simulink model "akh_rev_project"  (R2020b)
settings: Solver=ode45  StartTime=0.0  StopTime=10  FixedStep=Ts_Power  RelTol=1e-3  AbsTol=1e-2
InitFcn:
  | Fnom = 50;        % Hz
  | 
  | Fc = 27*Fnom;   % (Hz)
  | Ts_Power = 1/(Fc*100);
  | Ts_Control = Ts_Power*10;
values from neighbouring files (symbols this model uses):
  Ts = 1/fs    (= 1e-05)    [PE_46.m]    (also in disc_sim.m = 1; mass_spring_damper_model.m = 0.1)
undefined symbols (not defined in the file or in its folder): D1, D11, Delta, DiscIntNeverNeededParam, j, magnitude
libraries: powerlib x146, powerlib_meascontrol x90, simulink x2, re_lib x1
(part 2 of 8)

== system akh_rev_project/Source ==
  note: Adding negative-sequence and zero-sequence
      | 1 sec <  t < 1.5 sec
  note: Positive-sequence magnitude variation
  note: Vabc
      | Frequency Modulation
      |  58 /62 Hz
      |  Freq=1 Hz
  note: t = 1.75 sec
      | phase variation:
      | delta_phase= -60 deg
  note: t> 2 sec
      | Ajout d'harmoniques
      |  20% 3e  seq homopolaire
      |  30%  4e  seq directe
  -180 < alpha < 180 : Subsystem
  Bus Selector : BusSelector  OutputSignals=Freq (Hz)
  Bus Selector1 : BusSelector  OutputSignals=wt (rad)
  Mag (pu)2 : powerlib_meascontrol/Pulse & Signal Generators/Stair Generator  t="[0, 0.2, 0.3,  1]"  e="[1, 0.0,  1,  1.2]"  Ts=Ts
  Step : Step  Time=1.75  After=-90  SampleTime=0
  Sum : Sum  Inputs=+++
  Sum1 : Sum  Inputs=+-
  Synchronous Reference : powerlib_meascontrol/Pulse & Signal Generators/Three-Phase Programmable Generator  Par_Vps=[1, 0 , 60]  VariationEntity=None  VariationType=Modulation  VariationStep=-0.5  VariationRate=10  VariationMag=2  VariationFreq=1  Par_Timing_Variation="[0.5  99]"  SinglePhase=on  Yampli=[1 0.2 1.2 1.0]  Xtime=[0 0.1 0.15 0.2]  HarmonicGeneration=off  Par_HarmoA="[1  0.5  -25  0]"  Par_HarmoB="[1  0.1  35  2]"  Par_Timing_Harmo=[ 1 99]  Ts=Ts
      settings: SourceProductBaseCode=PS
  Terminator{,1..3} (4 alike) : Terminator
  Three-Phase Programmable Generator : powerlib_meascontrol/Pulse & Signal Generators/Three-Phase Programmable Generator  Par_Vps=[1, 0 , 60]  VariationEntity=Frequency  VariationType=Modulation  VariationStep=-0.5  VariationRate=10  VariationMag=2  VariationFreq=1  Par_Timing_Variation="[0.5  99]"  SinglePhase=on  Yampli=[1 0.2 1.2 1.0]  Xtime=[0 0.1 0.15 0.2]  HarmonicGeneration=off  Par_HarmoA="[1  0.5  -25  0]"  Par_HarmoB="[1  0.1  35  2]"  Par_Timing_Harmo=[ 1 99]  Ts=Ts
      settings: SourceProductBaseCode=PS
  Three-Phase Programmable Generator1 : powerlib_meascontrol/Pulse & Signal Generators/Three-Phase Programmable Generator  Par_Vps=[0 , 0 , 60]  VariationEntity=Frequency  VariationType=Modulation  VariationStep=-0.5  VariationRate=10  VariationMag=2  VariationFreq=1  Par_Timing_Variation="[0.5  99]"  SinglePhase=on  Yampli=[1 0.2 1.2 1.0]  Xtime=[0 0.1 0.15 0.2]  HarmonicGeneration=on  Par_HarmoA="[1  0.4  90  2]"  Par_HarmoB="[1  0.3  35  0]"  Par_Timing_Harmo=[1 1.5]  Ts=Ts
      settings: SourceProductBaseCode=PS
  Three-Phase Programmable Generator2 : powerlib_meascontrol/Pulse & Signal Generators/Three-Phase Programmable Generator  Par_Vps=[0 , 0 , 60]  VariationEntity=Frequency  VariationType=Modulation  VariationStep=-0.5  VariationRate=10  VariationMag=2  VariationFreq=1  Par_Timing_Variation="[0.5  99]"  SinglePhase=on  Yampli=[1 0.2 1.2 1.0]  Xtime=[0 0.1 0.15 0.2]  HarmonicGeneration=on  Par_HarmoA="[3  0.2  0  0]"  Par_HarmoB="[4  0.3  60  1]"  Par_Timing_Harmo="[ 2  99]"  Ts=Ts
      settings: SourceProductBaseCode=PS
  Three-Phase Sine Generator : powerlib_meascontrol/Pulse & Signal Generators/Three-Phase Sine Generator  Ts=Ts
      settings: SourceProductBaseCode=PS
  Vabc : Outport  VectorParamsAs1DForOutWhenUnconnected=off
  angle(deg) : Outport  Port=2  VectorParamsAs1DForOutWhenUnconnected=off
  tag scope: Freq_ref=global, Mag_ref=global
  wires:
  Step/1 -> Three-Phase Sine Generator/2
  Three-Phase Programmable Generator/2 -> Bus Selector/1
  Bus Selector/1 -> Three-Phase Sine Generator/3, [Freq_ref]  "<Freq (Hz)>"
  Mag (pu)2/1 -> [Mag_ref], Three-Phase Sine Generator/1
  Three-Phase Programmable Generator1/1 -> Sum/2
  Sum/1 -> Vabc/1  "Vabc (pu)"
  Three-Phase Programmable Generator2/1 -> Sum/3
  Three-Phase Sine Generator/1 -> Sum/1
  Three-Phase Programmable Generator/1 -> Terminator/1
  Three-Phase Programmable Generator2/2 -> Terminator1/1
  Three-Phase Programmable Generator1/2 -> Terminator2/1
  Bus Selector1/1 -> Sum1/2  "<wt (rad)>"
  Sum1/1 -> -180 < alpha < 180/1(angle (rad))
  Synchronous Reference/2 -> Bus Selector1/1
  Three-Phase Sine Generator/2 -> Sum1/1
  Synchronous Reference/1 -> Terminator3/1
  -180 < alpha < 180/1(angle(deg)) -> angle(deg)/1

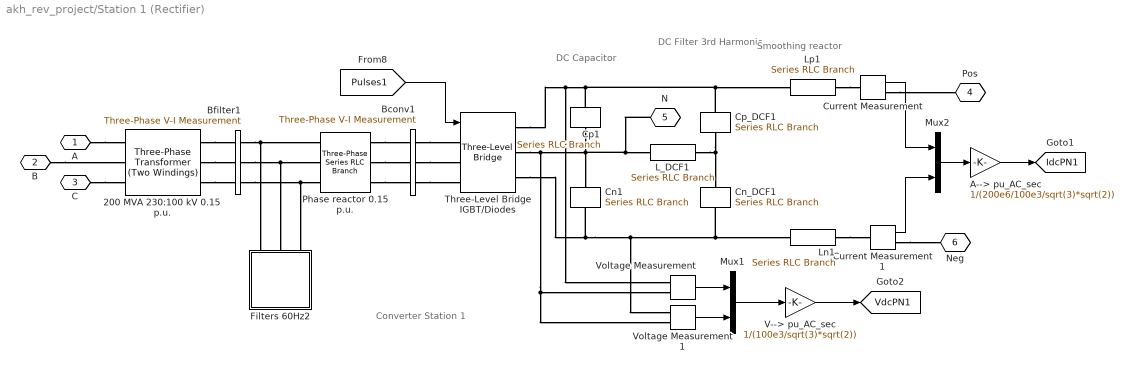
== system akh_rev_project/Station 1 (Rectifier) ==
  note: DC Capacitor
  note: Converter Station 1
  note: DC Filter
      | 3rd Harmonic
  note: Smoothing reactor
  200 MVA 230:100 kV 0.15 p.u. : powerlib/Elements/Three-Phase Transformer (Two Windings)  Winding1Connection=Yg  Winding2Connection=Delta (D1)  CoreType=Three single-phase transformers  SetSaturation=off  Hysteresis=off  DataFile='hysteresis'  SetInitialFlux=off  Measurements=None  UNITS=pu  NominalPower=[200e6 , Fnom]  Winding1="[230e3 * 0.915  0.0025 0.075]"  Winding2="[100e3  0.0025  0.075]"  Rm=500  Lm=500  L0=0.5  Saturation=[ 0,0 ; 0.012,1.25 ; 1.012,1.6 ]  InitialFluxes=[-1.03850588171453 0.527233233676132 0.511272648041703]  BreakLoop=off  DiscreteSolver=Trapezoidal iterative  DataType=off  TransfoNumber=0
  A--> pu_AC_sec : Gain  Gain=1/(200e6/100e3/sqrt(3)*sqrt(2))
  Bconv1 : powerlib/Measurements/Three-Phase V-I Measurement  VoltageMeasurement=phase-to-ground  SetLabelV=on  LabelV=Uv_abc1  Vpu=on  VpuLL=off  CurrentMeasurement=yes  SetLabelI=on  LabelI=Iv_abc1  Ipu=on  Pbase=200e6  Vbase=100e3  OutputType=Complex  PhasorSimulation=off  PSBequivalent=0
  Bfilter1 : powerlib/Measurements/Three-Phase V-I Measurement  VoltageMeasurement=phase-to-ground  SetLabelV=on  LabelV=Uf_abc1  Vpu=on  VpuLL=off  CurrentMeasurement=no  SetLabelI=off  LabelI=Iabc  Ipu=off  Pbase=100e6  Vbase=100e3  OutputType=Complex  PhasorSimulation=off  PSBequivalent=0
  Cn1 : powerlib/Elements/Series RLC Branch  LConnTagsString=__new0  RConnTagsString=__new0  BranchType=C  Resistance=[]  Inductance=[]  SetiL0=off  InitialCurrent=0  Capacitance=70e-6  Setx0=off  InitialVoltage=0  Measurements=None
  Cn_DCF1 : powerlib/Elements/Series RLC Branch  LConnTagsString=__new0  RConnTagsString=__new0  BranchType=C  Resistance=[]  Inductance=[]  SetiL0=off  InitialCurrent=0  Capacitance=12e-6  Setx0=off  InitialVoltage=0  Measurements=None
  Cp1 : powerlib/Elements/Series RLC Branch  LConnTagsString=__new0  RConnTagsString=__new0  BranchType=C  Resistance=[]  Inductance=[]  SetiL0=off  InitialCurrent=0  Capacitance=70e-6  Setx0=off  InitialVoltage=0  Measurements=None
  Cp_DCF1 : powerlib/Elements/Series RLC Branch  LConnTagsString=__new0  RConnTagsString=__new0  BranchType=C  Resistance=[]  Inductance=[]  SetiL0=off  InitialCurrent=0  Capacitance=12e-6  Setx0=off  InitialVoltage=0  Measurements=None
  Current Measurement : powerlib/Measurements/Current Measurement  PhasorSimulation=off  OutputType=Complex  PSBequivalent=0
  Current Measurement1 : powerlib/Measurements/Current Measurement  PhasorSimulation=off  OutputType=Complex  PSBequivalent=0
  Filters 60Hz2 : Subsystem
      mask Display: disp('AC filters\n40 Mvar')
  L_DCF1 : powerlib/Elements/Series RLC Branch  LConnTagsString=__new0  RConnTagsString=__new0  BranchType=RL  Resistance=0.14737  Inductance=46.908e-3  SetiL0=off  InitialCurrent=0  Capacitance=[]  Setx0=off  InitialVoltage=0  Measurements=None
  Ln1 : powerlib/Elements/Series RLC Branch  LConnTagsString=__new0  RConnTagsString=__new0  BranchType=RL  Resistance=0.0251  Inductance=8.0e-3  SetiL0=off  InitialCurrent=0  Capacitance=[]  Setx0=off  InitialVoltage=0  Measurements=Branch current
  Lp1 : powerlib/Elements/Series RLC Branch  LConnTagsString=__new0  RConnTagsString=__new0  BranchType=RL  Resistance=0.0251  Inductance=8.0e-3  SetiL0=off  InitialCurrent=0  Capacitance=[]  Setx0=off  InitialVoltage=0  Measurements=Branch current
  Mux1 : Mux  Inputs=2
  Mux2 : Mux  Inputs=2
  Phase reactor 0.15 p.u. : powerlib/Elements/Three-Phase Series RLC Branch  LConnTagsString=A|B|C  RConnTagsString=A|B|C  BranchType=RL  Resistance=0.0015*(100^2 / 200)  Inductance=0.15* (100^2 / 200) / (2*pi*Fnom)  Capacitance=1.0  Measurements=None
  Three-Level Bridge IGBT/Diodes : powerlib/Power Electronics/Three-Level Bridge  Arms=3  SnubberResistance=5000  SbubberCapacitance=1e-6  Device=IGBT / Diodes  Ron=1e-3  ForwardVoltages="[  0  0  ]"  Measurements=None
      settings: SourceProductBaseCode=PS
  V--> pu_AC_sec : Gain  Gain=1/(100e3/sqrt(3)*sqrt(2))
  Voltage Measurement : powerlib/Measurements/Voltage Measurement  PhasorSimulation=off  OutputType=Complex  PSBequivalent=0
  Voltage Measurement1 : powerlib/Measurements/Voltage Measurement  PhasorSimulation=off  OutputType=Complex  PSBequivalent=0
  A : PMIOPort  Side=Left
  B : PMIOPort  Port=2  Side=Left
  C : PMIOPort  Port=3  Side=Left
  Pos : PMIOPort  Tag=PMCPort  Port=4  Side=Right
  N : PMIOPort  Tag=PMCPort  Port=5  Side=Right
  Neg : PMIOPort  Tag=PMCPort  Port=6  Side=Right
  tag scope: IdcPN1=global, VdcPN1=global
  wires:
  [Pulses1] -> Three-Level Bridge IGBT/Diodes/1
  Current Measurement/1 -> Mux2/1
  Current Measurement1/1 -> Mux2/2
  Mux2/1 -> A--> pu_AC_sec/1
  Voltage Measurement/1 -> Mux1/1
  Voltage Measurement1/1 -> Mux1/2
  Mux1/1 -> V--> pu_AC_sec/1
  V--> pu_AC_sec/1 -> [VdcPN1]
  A--> pu_AC_sec/1 -> [IdcPN1]
  connections:
  A/RConn1 -- 200 MVA 230:100 kV 0.15 p.u./LConn1
  B/RConn1 -- 200 MVA 230:100 kV 0.15 p.u./LConn2
  C/RConn1 -- 200 MVA 230:100 kV 0.15 p.u./LConn3
  Phase reactor 0.15 p.u./RConn1 -- Bconv1/LConn1
  Phase reactor 0.15 p.u./RConn2 -- Bconv1/LConn2
  Phase reactor 0.15 p.u./RConn3 -- Bconv1/LConn3
  Bconv1/RConn1 -- Three-Level Bridge IGBT/Diodes/LConn1
  Bconv1/RConn2 -- Three-Level Bridge IGBT/Diodes/LConn2
  Bconv1/RConn3 -- Three-Level Bridge IGBT/Diodes/LConn3
  Cn1/RConn1 -- Three-Level Bridge IGBT/Diodes/RConn3 -- Voltage Measurement1/LConn1 -- Cn_DCF1/RConn1 -- Ln1/LConn1
  Cp_DCF1/LConn1 -- Three-Level Bridge IGBT/Diodes/RConn1 -- Voltage Measurement/LConn1 -- Cp1/LConn1 -- Lp1/LConn1
  Current Measurement/RConn1 -- Pos/RConn1
  Current Measurement1/RConn1 -- Neg/RConn1
  200 MVA 230:100 kV 0.15 p.u./RConn1 -- Bfilter1/LConn1
  200 MVA 230:100 kV 0.15 p.u./RConn2 -- Bfilter1/LConn2
  200 MVA 230:100 kV 0.15 p.u./RConn3 -- Bfilter1/LConn3
  Bfilter1/RConn2 -- Phase reactor 0.15 p.u./LConn2 -- Filters 60Hz2/LConn2
  Bfilter1/RConn3 -- Phase reactor 0.15 p.u./LConn3 -- Filters 60Hz2/LConn3
  Bfilter1/RConn1 -- Phase reactor 0.15 p.u./LConn1 -- Filters 60Hz2/LConn1
  Cp_DCF1/RConn1 -- Cn_DCF1/LConn1 -- L_DCF1/RConn1
  N/RConn1 -- Voltage Measurement/LConn2 -- Voltage Measurement1/LConn2 -- Three-Level Bridge IGBT/Diodes/RConn2 -- Cn1/LConn1 -- Cp1/RConn1 -- L_DCF1/LConn1
  Lp1/RConn1 -- Current Measurement/LConn1
  Ln1/RConn1 -- Current Measurement1/LConn1

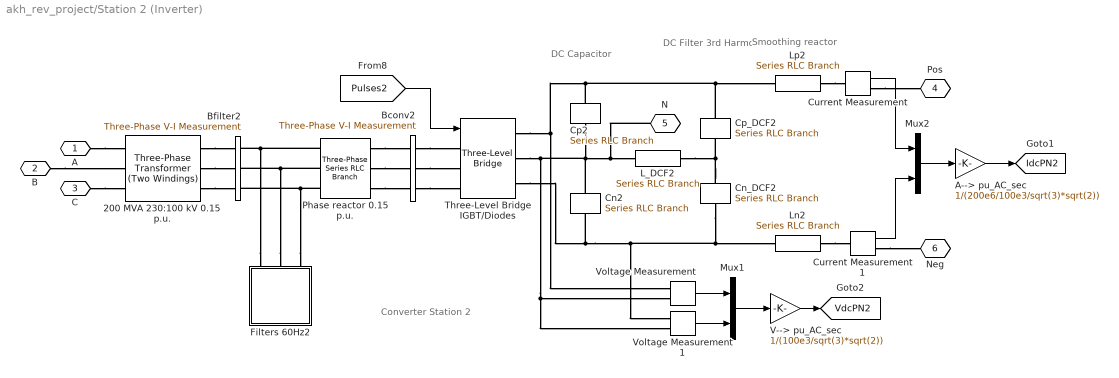
== system akh_rev_project/Station 2 (Inverter) ==
  note: Converter Station 2
  note: DC Capacitor
  note: DC Filter
      | 3rd Harmonic
  note: Smoothing reactor
  200 MVA 230:100 kV 0.15 p.u. : powerlib/Elements/Three-Phase Transformer (Two Windings)  Winding1Connection=Yg  Winding2Connection=Delta (D1)  CoreType=Three single-phase transformers  SetSaturation=off  Hysteresis=off  DataFile='hysteresis'  SetInitialFlux=off  Measurements=None  UNITS=pu  NominalPower=[200e6 , Fnom]  Winding1="[230e3 * 1.015   0.0025  0.075]"  Winding2="[100e3  0.0025  0.075]"  Rm=500  Lm=500  L0=0.5  Saturation=[ 0,0 ; 0.012,1.25 ; 1.012,1.6 ]  InitialFluxes=[-1.00735070526646 0.511416236666093 0.495934468600514]  BreakLoop=off  DiscreteSolver=Trapezoidal iterative  DataType=off  TransfoNumber=0
  A--> pu_AC_sec : Gain  Gain=1/(200e6/100e3/sqrt(3)*sqrt(2))
  Bconv2 : powerlib/Measurements/Three-Phase V-I Measurement  VoltageMeasurement=phase-to-ground  SetLabelV=on  LabelV=Uv_abc2  Vpu=on  VpuLL=off  CurrentMeasurement=yes  SetLabelI=on  LabelI=Iv_abc2  Ipu=on  Pbase=200e6  Vbase=100e3  OutputType=Complex  PhasorSimulation=off  PSBequivalent=0
  Bfilter2 : powerlib/Measurements/Three-Phase V-I Measurement  VoltageMeasurement=phase-to-ground  SetLabelV=on  LabelV=Uf_abc2  Vpu=on  VpuLL=off  CurrentMeasurement=no  SetLabelI=off  LabelI=Iabc  Ipu=off  Pbase=100e6  Vbase=100e3  OutputType=Complex  PhasorSimulation=off  PSBequivalent=0
  Cn2 : powerlib/Elements/Series RLC Branch  LConnTagsString=__new0  RConnTagsString=__new0  BranchType=C  Resistance=[]  Inductance=[]  SetiL0=off  InitialCurrent=0  Capacitance=70e-6  Setx0=off  InitialVoltage=0  Measurements=None
  Cn_DCF2 : powerlib/Elements/Series RLC Branch  LConnTagsString=__new0  RConnTagsString=__new0  BranchType=C  Resistance=[]  Inductance=[]  SetiL0=off  InitialCurrent=0  Capacitance=12e-6  Setx0=off  InitialVoltage=0  Measurements=None
  Cp2 : powerlib/Elements/Series RLC Branch  LConnTagsString=__new0  RConnTagsString=__new0  BranchType=C  Resistance=[]  Inductance=[]  SetiL0=off  InitialCurrent=0  Capacitance=70e-6  Setx0=off  InitialVoltage=0  Measurements=None
  Cp_DCF2 : powerlib/Elements/Series RLC Branch  LConnTagsString=__new0  RConnTagsString=__new0  BranchType=C  Resistance=[]  Inductance=[]  SetiL0=off  InitialCurrent=0  Capacitance=12e-6  Setx0=off  InitialVoltage=0  Measurements=None
  Current Measurement : powerlib/Measurements/Current Measurement  PhasorSimulation=off  OutputType=Complex  PSBequivalent=0
  Current Measurement1 : powerlib/Measurements/Current Measurement  PhasorSimulation=off  OutputType=Complex  PSBequivalent=0
  Filters 60Hz2 : Subsystem
      mask Display: disp('AC filters\n40 Mvar')
  L_DCF2 : powerlib/Elements/Series RLC Branch  LConnTagsString=__new0  RConnTagsString=__new0  BranchType=RL  Resistance=0.14737  Inductance=46.908e-3  SetiL0=off  InitialCurrent=0  Capacitance=[]  Setx0=off  InitialVoltage=0  Measurements=None
  Ln2 : powerlib/Elements/Series RLC Branch  LConnTagsString=__new0  RConnTagsString=__new0  BranchType=RL  Resistance=0.0251  Inductance=8.0e-3  SetiL0=off  InitialCurrent=0  Capacitance=[]  Setx0=off  InitialVoltage=0  Measurements=Branch current
  Lp2 : powerlib/Elements/Series RLC Branch  LConnTagsString=__new0  RConnTagsString=__new0  BranchType=RL  Resistance=0.0251  Inductance=8.0e-3  SetiL0=off  InitialCurrent=0  Capacitance=[]  Setx0=off  InitialVoltage=0  Measurements=Branch current
  Mux1 : Mux  Inputs=2
  Mux2 : Mux  Inputs=2
  Phase reactor 0.15 p.u. : powerlib/Elements/Three-Phase Series RLC Branch  LConnTagsString=A|B|C  RConnTagsString=A|B|C  BranchType=RL  Resistance=(0.15/100)*(100^2 / 200)  Inductance=0.15 * (100^2 / 200) / (2*pi*Fnom)  Capacitance=1.0  Measurements=None
  Three-Level Bridge IGBT/Diodes : powerlib/Power Electronics/Three-Level Bridge  Arms=3  SnubberResistance=5000  SbubberCapacitance=1e-6  Device=IGBT / Diodes  Ron=1e-3  ForwardVoltages="[ 0  0  ]"  Measurements=None
      settings: SourceProductBaseCode=PS
  V--> pu_AC_sec : Gain  Gain=1/(100e3/sqrt(3)*sqrt(2))
  Voltage Measurement : powerlib/Measurements/Voltage Measurement  PhasorSimulation=off  OutputType=Complex  PSBequivalent=0
  Voltage Measurement1 : powerlib/Measurements/Voltage Measurement  PhasorSimulation=off  OutputType=Complex  PSBequivalent=0
  A : PMIOPort  Side=Left
  B : PMIOPort  Port=2  Side=Left
  C : PMIOPort  Port=3  Side=Left
  Pos : PMIOPort  Tag=PMCPort  Port=4  Side=Right
  N : PMIOPort  Tag=PMCPort  Port=5  Side=Right
  Neg : PMIOPort  Tag=PMCPort  Port=6  Side=Right
  tag scope: IdcPN2=global, VdcPN2=global
  wires:
  Mux1/1 -> V--> pu_AC_sec/1
  Voltage Measurement1/1 -> Mux1/2
  Voltage Measurement/1 -> Mux1/1
  Mux2/1 -> A--> pu_AC_sec/1
  Current Measurement1/1 -> Mux2/2
  Current Measurement/1 -> Mux2/1
  [Pulses2] -> Three-Level Bridge IGBT/Diodes/1
  A--> pu_AC_sec/1 -> [IdcPN2]
  V--> pu_AC_sec/1 -> [VdcPN2]
  connections:
  Filters 60Hz2/LConn1 -- Bfilter2/RConn1 -- Phase reactor 0.15 p.u./LConn1
  Filters 60Hz2/LConn3 -- Bfilter2/RConn3 -- Phase reactor 0.15 p.u./LConn3
  Filters 60Hz2/LConn2 -- Bfilter2/RConn2 -- Phase reactor 0.15 p.u./LConn2
  200 MVA 230:100 kV 0.15 p.u./RConn3 -- Bfilter2/LConn3
  200 MVA 230:100 kV 0.15 p.u./RConn2 -- Bfilter2/LConn2
  200 MVA 230:100 kV 0.15 p.u./RConn1 -- Bfilter2/LConn1
  Current Measurement1/RConn1 -- Neg/RConn1
  Current Measurement/RConn1 -- Pos/RConn1
  Cp_DCF2/LConn1 -- Three-Level Bridge IGBT/Diodes/RConn1 -- Voltage Measurement/LConn1 -- Cp2/LConn1 -- Lp2/LConn1
  Cn_DCF2/RConn1 -- Voltage Measurement1/LConn1 -- Three-Level Bridge IGBT/Diodes/RConn3 -- Cn2/RConn1 -- Ln2/LConn1
  Cn2/LConn1 -- Voltage Measurement1/LConn2 -- Voltage Measurement/LConn2 -- Three-Level Bridge IGBT/Diodes/RConn2 -- Cp2/RConn1 -- L_DCF2/LConn1 -- N/RConn1
  Bconv2/RConn3 -- Three-Level Bridge IGBT/Diodes/LConn3
  Bconv2/RConn2 -- Three-Level Bridge IGBT/Diodes/LConn2
  Bconv2/RConn1 -- Three-Level Bridge IGBT/Diodes/LConn1
  Phase reactor 0.15 p.u./RConn3 -- Bconv2/LConn3
  Phase reactor 0.15 p.u./RConn2 -- Bconv2/LConn2
  Phase reactor 0.15 p.u./RConn1 -- Bconv2/LConn1
  C/RConn1 -- 200 MVA 230:100 kV 0.15 p.u./LConn3
  B/RConn1 -- 200 MVA 230:100 kV 0.15 p.u./LConn2
  A/RConn1 -- 200 MVA 230:100 kV 0.15 p.u./LConn1
  Cn_DCF2/LConn1 -- Cp_DCF2/RConn1 -- L_DCF2/RConn1
  Lp2/RConn1 -- Current Measurement/LConn1
  Ln2/RConn1 -- Current Measurement1/LConn1

== system akh_rev_project/VSC Controller Station 1 ==
  note: |-----------------------Ts_Control-----------------------|
  note: |------------Ts_Power------------|
  note: Sample time:
  note: |----------------Ts_Power--------------|
  note: Reference Steps
  note: VSC Controller
      | (Station 1)
  Anti-aliasing Filters : Subsystem  mask(Anti-aliasing (2nd order lowpass)){f0_aa=2000, Ts=Ts_Power}
      mask prompts: f0_aa "Cut-off frequency (Hz):"; Ts "Sample time:"
      mask init:
      | zeta = 1/sqrt(2);
  Block : Step  Time=0.3  Before=1  After=0  SampleTime=Ts_Control
  Constant1 : Constant  Value=0
  Constant2 : Constant  Value=0
  Constant3 : Constant  Value=1.0
  "Discrete VSC Controller " : Subsystem  mask(Discrete VSC-Based HVDC Controller){Mode=Active & Reactive Power, Xnom=[230e3, 100e3, Fnom, 200e3, 200e6], XP=[20.0, 1.0, -1.0, 1.43], Xdvco=[3.0, 3.0, 1.05, 0.9], XUdc=[2.0, 40.0 ], XQ=[20.0, 0.5, -0.5], Xvco=[3.0, 3.0, 1.05, 0.94], Xcrc=[1.1,  0.8], Xaccc=[0.6, 6.0,  0.3], enable_dcvbc=off, Xdcvbc=[0.2, 0.03], Ts_Control=Ts_Control}
      mask prompts: Mode "Control Mode:"; Xnom "Nominal AC & DC values: [ Vpcc(Vrms L-L) , Vconv (Vrms L-L),  Freq. (Hz), Vdc (V L-L), Pnom (VA) ]"; XP "P Regulator [ Ki (1/s), Pmax (pu), Pmin (pu), Ramp (pu/s)]"; Xdvco "P Control: Udc Override [ Kp, Ki (1/s), Udc_max (pu), Udc_min (pu)]"; XUdc "DC Voltage Regulator [ Kp, Ki (1/s)]"; XQ "Q Regulator [ Ki (1/s), Qmax (pu), Qmin (pu)]"; Xvco "Q Control: Uac Override [ Kp, Ki (1/s), U_max (pu), U_min (pu)]"; Xcrc "Current Reference Limits [ lim_d (pu),  lim_q (pu)]"; Xaccc "Inner Current Regulator [ Kp, Ki (1/s), Kf (pu)]"; enable_dcvbc "DC Voltage Balance"; Xdcvbc "DC Voltage Balance Control} [ Kp, Ki (1/s)]"; Ts_Control "Sample Time (s)"
      mask help:
      | This block implements a controller for a VSC (Voltage-Sourced Converter) HVDC using a three-level or Neutral Point Clamped (NPC) converter bridge.
      | The 'Vref_abc' output contains the three modulating signals used by  the carrier-based  Sinusoidal Pulse Width Modulation (SPWM) pulse generator.
      | The output  'm' is a bus signal . Use the Bus Selector block to extract individual signals.
      |
      | See the "VSC-Based Transmission Link " tutorial for a description of the control system.
      mask init:
      | if (Mode == 1)
      | 	P_control = 1;
      | else
      | 	P_control = 0;
      | end
      | 	
      | % Nominal AC & DC values:
      | VacNom1 = Xnom(1); VacNom2 = Xnom(2); Fnom = Xnom(3);
      | VdcNom = Xnom(4); Pnom = Xnom(5);
      | % Normalisation Calculation
      | Uac_sec_to_pu   = 1/(VacNom2*sqrt(2)/sqrt(3));      % Vrms(L-L) ==> pu Vac
      | k_nom2pu_Vdc = (VdcNom/2) * Uac_sec_to_pu;          % pu Vdc ==> pu Vac    
      | k_pu2nom_Vdc = 1/k_nom2pu_Vdc;                      % pu Vac ==> pu Vdc
      | k_nom2pu_Idc = ((VacNom2)*sqrt(3))/(sqrt(2)*VdcNom);% pu Idc ==> pu Iac
      | k_pu2nom_Idc = 1/k_nom2pu_Idc;                      % pu Iac ==> pu Idc
      | % Transformer connexion:
      | Tr_connection = 1;
      | % P regulator:
      | Ki_apc = XP(1); P_max = XP(2); P_min = XP(3); Ramp_apc = XP(4);
      | max_i_apc = 10; min_i_apc = -max_i_apc; V_level_apc = 0.9;  % (pu)
      | % DC Voltage Control Override:
      | Ki_apc_vco = Xdvco(2); Kp_apc_vco = Xdvco(1);
      | Udc_max = Xdvco(3)*k_nom2pu_Vdc; Udc_min = Xdvco(4)*k_nom2pu_Vdc;
      | max_apc_vco = 1.0; min_apc_vco = -max_apc_vco;
      | % Q regulator:
      | Ki_rpc = XQ(1);Q_max = XQ(2); Q_min = XQ(3);
      | max_i_rpc = 10; min_i_rpc = -max_i_rpc; V_level_rpc = 0.9;  % (pu)
      | % AC Voltage Control Override:
      | Ki_rpc_vco = Xvco(2); Kp_rpc_vco = Xvco(1);
      | U_max = Xvco(3); U_min = Xvco(4);
      | max_rpc_vco = 1.0; min_rpc_vco = -max_rpc_vco;
      | % Current Reference Calculation:
      | lim_d_crc = Xcrc(1); lim_q_crc = Xcrc(2); %(pu)
      | U_level_crc = 0.7; %(pu)
      | f0_crc = 100; % (Hz)
      | % Current Reference Limitation:
      | Iref_max = sqrt(lim_d_crc^2 + lim_q_crc^2);
      | % DC Voltage regulator:
      | Ki_dcvc = XUdc(2); Kp_dcvc = XUdc(1);
      | max_i_dcvc = lim_d_crc; min_i_dcvc = -max_i_dcvc;
      | max_out_dcvc = max_i_dcvc; min_out_dcvc = -max_out_dcvc; % (pu)
      | f0_Udc = 10.0; % (Hz)
      | % Inner Current Loop:
      | Ki_accc = Xaccc(2); Kp_accc = Xaccc(1); Kf_accc = Xaccc(3);
      | max_out_accc = 2.0; min_out_accc = -max_out_accc;
      | %PLL
      | f_min_pll = 0.75*Fnom; % (Hz)
      | Kp_pll = 60.0;
      | Ki_pll = 1400;
      | % Inner Current Loop:
      | K_pwm = 1.0; 
      | % DC Voltage Balance Control:
      | Ki_dcvbc = Xdcvbc(2); Kp_dcvbc = Xdcvbc(1);
      | f0_dcvbc =  1.0;   % (Hz)
      | max_out_dcvbc = 0.2; min_out_dcvbc = -max_out_dcvbc;
      | % Signal Calculations:
      | f0_sc = 17; %(Hz)
      | zeta_sc = 1/sqrt(2);
      mask TypeOptions Mode: Active & Reactive Power | DC Voltage & Reactive  Power
      mask Callback Mode:
      | tempMaskVis=get_param(gcb,'MaskVisibilities');
      | if strcmp(get_param(gcb,'Mode'),'Active & Reactive Power')
      | 	tempMaskVis{2}='on'; tempMaskVis{3}='on'; tempMaskVis{4}='on'; tempMaskVis{5}='on';
      | 	tempMaskVis{6}='on'; tempMaskVis{5}='off'; tempMaskVis{8}='on'; tempMaskVis{9}='on';
      | 	tempMaskVis{10}='on';  tempMaskVis{12}='on';
      | 
      | else
      | 	tempMaskVis{2}='on'; tempMaskVis{3}='off'; tempMaskVis{4}='off'; tempMaskVis{5}='on';
      | 	tempMaskVis{6}='on'; tempMaskVis{7}='on'; tempMaskVis{8}='on'; tempMaskVis{9}='on';
      | 	tempMaskVis{10}='on';  tempMaskVis{12}='on';
      | end
      | if strcmp(get_param(gcb,'enable_dcvbc'),'on')
      | 	tempMaskVis{11}='on';
      | else
      | 	tempMaskVis{11}='off';
      | end
      | set_param(gcb,'MaskVisibilities',tempMaskVis);
      mask Callback enable_dcvbc:
      | tempMaskVis=get_param(gcb,'MaskVisibilities');
      | if strcmp(get_param(gcb,'enable_dcvbc'),'on')
      | 	tempMaskVis{11}='on';
      | else
      | 	tempMaskVis{11}='off';
      | end
      | set_param(gcb,'MaskVisibilities',tempMaskVis);
  PWM Generator (3-Level) : powerlib_meascontrol/Pulse & Signal Generators/PWM Generator (3-Level)  ModulatorType=Three-phase bridge (12 pulses)  ModulatorMode=Unsynchronized  nF=27  Fc=27*Fnom  ModulatingSignals=off  m=0.8  Freq=60  Phase=0  Ts=Ts_Power
      settings: SourceProductBaseCode=PS
  Pref : Step  Time=1.5 * 1  After=-0.1  SampleTime=Ts_Control
  Qref : Step  Time=2.0 * 1  After=-0.1  SampleTime=Ts_Control
  Switch : Switch  Criteria=u2 > Threshold  SaturateOnIntegerOverflow=on
  Unit Delay : UnitDelay  SampleTime=Ts_Control  HasFrameUpgradeWarning=on
  Zero-Order Hold{1..3,5,7,13} (6 alike) : ZeroOrderHold  SampleTime=Ts_Control
  tag scope: Control1=global, Pulses1=global, Qref1=global, Udref1=global, Vref_abc1=global
  wires:
  "Discrete VSC Controller "/1(Vref_abc) -> Unit Delay/1, [Vref_abc1]
  Zero-Order Hold13/1 -> "Discrete VSC Controller "/1(Uabc (pu))
  Zero-Order Hold1/1 -> "Discrete VSC Controller "/2(Iabc (pu))
  Zero-Order Hold3/1 -> "Discrete VSC Controller "/3(Uf_abc (pu))
  Zero-Order Hold2/1 -> "Discrete VSC Controller "/4(Iv_abc (pu))
  Zero-Order Hold5/1 -> "Discrete VSC Controller "/5(Udc_pn (pu))
  Zero-Order Hold7/1 -> "Discrete VSC Controller "/6(Idc_pn (pu))
  [Iabc_B1] -> Anti-aliasing Filters/2("Iabc ")
  [Uf_abc1] -> Anti-aliasing Filters/3("Uf_abc  ")
  [Iv_abc1] -> Anti-aliasing Filters/4("Iv_abc ")
  Anti-aliasing Filters/2(Iabc) -> Zero-Order Hold1/1
  Anti-aliasing Filters/3(Uf_abc) -> Zero-Order Hold3/1
  Anti-aliasing Filters/4(" Iv_abc") -> Zero-Order Hold2/1
  Anti-aliasing Filters/5("Udc_pn ") -> Zero-Order Hold5/1
  Anti-aliasing Filters/6(" Idc_pn") -> Zero-Order Hold7/1
  Unit Delay/1 -> PWM Generator (3-Level)/1
  Switch/1 -> [Pulses1]
  Constant2/1 -> Switch/1
  Constant1/1 -> "Discrete VSC Controller "/10(Udref), [Udref1]
  Qref/1 -> "Discrete VSC Controller "/9(Qref), [Qref1]
  Pref/1 -> "Discrete VSC Controller "/8(dPref)
  Constant3/1 -> "Discrete VSC Controller "/7(Pref)
  Block/1 -> Switch/2, "Discrete VSC Controller "/11(block_status)
  [VdcPN1] -> Anti-aliasing Filters/5("Udc_pn  ")
  [IdcPN1] -> Anti-aliasing Filters/6("Idc_pn ")
  "Discrete VSC Controller "/2(m) -> [Control1]
  [Uabc_B1] -> Anti-aliasing Filters/1("Uabc ")
  Anti-aliasing Filters/1(Uabc) -> Zero-Order Hold13/1
  PWM Generator (3-Level)/1 -> Switch/3

== system akh_rev_project/VSC Controller Station 2 ==
  note: VSC Controller
      | (Station 2)
  note: |----------------Ts_Power--------------|
  note: Sample time:
  note: |------------Ts_Power------------|
  note: |---------------------------Ts_Control-------------------------|
  note: Reference Steps
  Anti-aliasing Filters : Subsystem  mask(Anti-aliasing (2nd order lowpass)){f0_aa=2000, Ts=Ts_Power}
      mask prompts: f0_aa "Cut-off frequency (Hz):"; Ts "Sample time:"
      mask init:
      | zeta = 1/sqrt(2);
  Block : Step  Time=0.1  Before=1  After=0  SampleTime=Ts_Control
  Constant1 : Constant  Value=0
  Constant2 : Constant  Value=0
  Constant3 : Constant  Value=0
  Constant4 : Constant  Value=-0.1
  "Discrete VSC Controller " : Subsystem  mask(Discrete VSC-Based HVDC Controller){Mode=DC Voltage & Reactive  Power, Xnom=[230e3, 100e3, Fnom, 200e3, 200e6], XP=[20.0, 1.0, -1.0, 1.43], Xdvco=[3.0, 3.0, 1.05, 0.9], XUdc=[2.0, 40.0 ], XQ=[20.0, 0.5, -0.5], Xvco=[3.0, 3.0, 1.05, 0.94], Xcrc=[1.1,  0.8], Xaccc=[0.6, 6.0,  0.3], enable_dcvbc=on, Xdcvbc=[0.2, 0.03], Ts_Control=Ts_Control}
      mask prompts: Mode "Control Mode:"; Xnom "Nominal AC & DC values: [ Vpcc(Vrms L-L) , Vconv (Vrms L-L),  Freq. (Hz), Vdc (V L-L), Pnom (VA) ]"; XP "P Regulator [ Ki (1/s), Pmax (pu), Pmin (pu), Ramp (pu/s)]"; Xdvco "P Control: Udc Override [ Kp, Ki (1/s), Udc_max (pu), Udc_min (pu)]"; XUdc "DC Voltage Regulator [ Kp, Ki (1/s)]"; XQ "Q Regulator [ Ki (1/s), Qmax (pu), Qmin (pu)]"; Xvco "Q Control: Uac Override [ Kp, Ki (1/s), U_max (pu), U_min (pu)]"; Xcrc "Current Reference Limits [ lim_d (pu),  lim_q (pu)]"; Xaccc "Inner Current Regulator [ Kp, Ki (1/s), Kf (pu)]"; enable_dcvbc "DC Voltage Balance"; Xdcvbc "DC Voltage Balance Control} [ Kp, Ki (1/s)]"; Ts_Control "Sample Time (s)"
      mask help:
      | This block implements a controller for a VSC (Voltage-Sourced Converter) HVDC using a three-level or Neutral Point Clamped (NPC) converter bridge.
      | The 'Vref_abc' output contains the three modulating signals used by  the carrier-based  Sinusoidal Pulse Width Modulation (SPWM) pulse generator.
      | The output  'm' is a bus signal . Use the Bus Selector block to extract individual signals.
      |
      | See the "VSC-Based Transmission Link " tutorial for a description of the control system.
      mask init: same as akh_rev_project/VSC Controller Station 1/Discrete VSC Controller 
      mask TypeOptions Mode: Active & Reactive Power | DC Voltage & Reactive  Power
      mask Callback Mode:
      | tempMaskVis=get_param(gcb,'MaskVisibilities');
      | if strcmp(get_param(gcb,'Mode'),'Active & Reactive Power')
      | 	tempMaskVis{2}='on'; tempMaskVis{3}='on'; tempMaskVis{4}='on'; tempMaskVis{5}='on';
      | 	tempMaskVis{6}='on'; tempMaskVis{5}='off'; tempMaskVis{8}='on'; tempMaskVis{9}='on';
      | 	tempMaskVis{10}='on';  tempMaskVis{12}='on';
      | 
      | else
      | 	tempMaskVis{2}='on'; tempMaskVis{3}='off'; tempMaskVis{4}='off'; tempMaskVis{5}='on';
      | 	tempMaskVis{6}='on'; tempMaskVis{7}='on'; tempMaskVis{8}='on'; tempMaskVis{9}='on';
      | 	tempMaskVis{10}='on';  tempMaskVis{12}='on';
      | end
      | if strcmp(get_param(gcb,'enable_dcvbc'),'on')
      | 	tempMaskVis{11}='on';
      | else
      | 	tempMaskVis{11}='off';
      | end
      | set_param(gcb,'MaskVisibilities',tempMaskVis);
      mask Callback enable_dcvbc:
      | tempMaskVis=get_param(gcb,'MaskVisibilities');
      | if strcmp(get_param(gcb,'enable_dcvbc'),'on')
      | 	tempMaskVis{11}='on';
      | else
      | 	tempMaskVis{11}='off';
      | end
      | set_param(gcb,'MaskVisibilities',tempMaskVis);
  PWM Generator (3-Level) : powerlib_meascontrol/Pulse & Signal Generators/PWM Generator (3-Level)  ModulatorType=Three-phase bridge (12 pulses)  ModulatorMode=Unsynchronized  nF=27  Fc=27*Fnom  ModulatingSignals=off  m=0.8  Freq=60  Phase=0  Ts=Ts_Power
      settings: SourceProductBaseCode=PS
  Switch : Switch  Criteria=u2 > Threshold  SaturateOnIntegerOverflow=on
  Udref : Step  Time=2.5 * 1  Before=1.0  After=0.95  SampleTime=Ts_Control
  Unit Delay : UnitDelay  SampleTime=Ts_Control  HasFrameUpgradeWarning=on
  tag scope: Control2=global, Pulses2=global, Qref2=global, Udref2=global, Vref_abc2=global
  wires:
  Block/1 -> Switch/2, "Discrete VSC Controller "/11(block_status)
  Constant2/1 -> Switch/1
  Switch/1 -> [Pulses2]
  Unit Delay/1 -> PWM Generator (3-Level)/1
  [Iv_abc2] -> Anti-aliasing Filters/4("Iv_abc ")
  [Uf_abc2] -> Anti-aliasing Filters/3("Uf_abc  ")
  [Iabc_B2] -> Anti-aliasing Filters/2("Iabc ")
  [Uabc_B2] -> Anti-aliasing Filters/1("Uabc ")
  [VdcPN2] -> Anti-aliasing Filters/5("Udc_pn  ")
  [IdcPN2] -> Anti-aliasing Filters/6("Idc_pn ")
  Anti-aliasing Filters/1(Uabc) -> "Discrete VSC Controller "/1(Uabc (pu))
  Anti-aliasing Filters/2(Iabc) -> "Discrete VSC Controller "/2(Iabc (pu))
  Anti-aliasing Filters/3(Uf_abc) -> "Discrete VSC Controller "/3(Uf_abc (pu))
  Anti-aliasing Filters/4(" Iv_abc") -> "Discrete VSC Controller "/4(Iv_abc (pu))
  Anti-aliasing Filters/5("Udc_pn ") -> "Discrete VSC Controller "/5(Udc_pn (pu))
  Anti-aliasing Filters/6(" Idc_pn") -> "Discrete VSC Controller "/6(Idc_pn (pu))
  Constant3/1 -> "Discrete VSC Controller "/7(Pref)
  Constant4/1 -> "Discrete VSC Controller "/9(Qref), [Qref2]
  Udref/1 -> "Discrete VSC Controller "/10(Udref), [Udref2]
  Constant1/1 -> "Discrete VSC Controller "/8(dPref)
  "Discrete VSC Controller "/2(m) -> [Control2]
  "Discrete VSC Controller "/1(Vref_abc) -> Unit Delay/1, [Vref_abc2]
  PWM Generator (3-Level)/1 -> Switch/3

== system akh_rev_project/AC System 1/Measurements ==
  Grid : Scope  NumInputPorts=8
  Grid Data acquisition : Subsystem
  Wind Turbine : Scope  NumInputPorts=8
  Wind turbine Data acquisition : Subsystem
  wires:
  Wind turbine Data acquisition/3(P_mean) -> Wind Turbine/3  "Generated P(MW)"
  Grid Data acquisition/1("Vabc_B120 ") -> Grid/1  "Vabc_B120 (pu)"
  Grid Data acquisition/2("Vabc_B25 ") -> Grid/2  "Vabc_B25 (pu)"
  Grid Data acquisition/3("Vabc_B575 ") -> Grid/3  "Vabc_B575 (pu)"
  Grid Data acquisition/4(P_B25) -> Grid/4  "P_B25 (MW)"
  Grid Data acquisition/5(Q_B25) -> Grid/5  "Q_B25 (Mvar)"
  [Vdc] -> Wind Turbine/5  "Vdc (V)"
  [wr] -> Wind Turbine/6  "Speed (pu)"
  Wind turbine Data acquisition/1(V1_B575) -> Wind Turbine/1  "Pos. seq. V1_B575 (pu)"
  Wind turbine Data acquisition/2(I1_B575) -> Wind Turbine/2  "Pos. seq. I1_B575 (pu)"
  Wind turbine Data acquisition/4(Q_mean) -> Wind Turbine/4  "Generated Q(Mvar)"
  Grid Data acquisition/8(Motor_Speed) -> Grid/8  "Motor Speed (pu)"
  Grid Data acquisition/7(I1_Plant) -> Grid/7  "I Plant pos. seq. (pu/2 MVA)"
  Grid Data acquisition/6(V1_Plant) -> Grid/6  "V_Plant 2.3kV pos. seq. (pu)"
  [wind] -> Wind Turbine/7  "Wind speed (m/s)"
  [pitch] -> Wind Turbine/8  "pitch angle (deg)"

== system akh_rev_project/AC System 1/More info ==

== system akh_rev_project/AC System 1/Plant 2 MVA ==
  note: Instantaneous AC Overcurrent
  note: AC Overcurrent (positive-sequence)
  note: AC Current Unbalance
  note: AC Undervoltage (positive-sequence)
  note: AC Overvoltage (positive-sequence)
  note: AC Voltage Unbalance (Negative-sequence)
  note: AC Voltage Unbalance (Zero-sequence)
  note: DC Overvoltage
  note: Under Speed
  note: Over Speed
  1.68 MW 0.93 PF 2300 V : powerlib/Machines/Asynchronous Machine pu Units  RotorType=Squirrel-cage  PresetModel=No  MechanicalLoad=Torque Tm  ShowDetailedParameters=on  ReferenceFrame=Rotor  Units=pu  MeasurementBus=off  NominalParameters=[1.68e6/0.93 2300 60]  Stator=[0.0092 0.0717]  Rotor=[0.007 0.0717]  Cage1=[0.01909 0.0397]  Cage2=[0.01909 0.0397]  Lm=4.14  Mechanical=[0.5 0 2]  PolePairs=2  InitialConditions="[ 1e-3,0   0,0,0   0,0,0 ]"  SimulateSaturation=off  Saturation=[ 0 0 ; 0 0 ]  LoadFlowParameters=0  TsPowergui=0  TsBlock=-1  IterativeModel=Forward Euler  IterativeDiscreteModel=Trapezoidal non iterative  Pmec=3e3
      settings: SourceProductBaseCode=PS
  200 kW : powerlib/Elements/Three-Phase Series RLC Load  LConnTagsString=A|B|C  Configuration=Y (grounded)  NominalVoltage=2300  Vabc=[1e3 1e3 1e3]  Vabcp=[1e3 1e3 1e3]  NominalFrequency=60  UnbalancedPower=off  ActivePower=200e3  InductivePower=0  CapacitivePower=0  Pabc=[10e3 9e3 11e3]  QLabc=[100 90 110]  QCabc=[100 90 110]  Pabcp=[10e3 9e3 11e3]  QLabcp=[100 90 110]  QCabcp=[100 90 110]  Measurements=None  LoadType=constant Z
  25/2.3 kV 2.5 MVA : powerlib/Elements/Three-Phase Transformer (Two Windings)  Winding1Connection=Delta (D11)  Winding2Connection=Yn  CoreType=Three single-phase transformers  SetSaturation=off  Hysteresis=off  DataFile='basic_model'  SetInitialFlux=off  Measurements=None  UNITS=pu  NominalPower=[2.5e6 60 ]  Winding1="[ 25e3  0.04/30   0.04 ]"  Winding2="[ 2.3e3  0.04/30  0.04]"  Rm=500  Lm=500  L0=0.5  Saturation="[ 0,0  ;  0.005,1.2  ;  1.0,1.4 ]"  InitialFluxes=[ 0.8 , -0.8 , 0.7 ]  BreakLoop=off  DiscreteSolver=Trapezoidal iterative  DataType=off  TransfoNumber=0
  265 ohms : powerlib/Elements/Series RLC Branch  LConnTagsString=__new0  RConnTagsString=__new0  BranchType=R  Resistance=265  Inductance=1.0  SetiL0=off  InitialCurrent=0  Capacitance=1.0  Setx0=off  InitialVoltage=0  Measurements=None
  B2300 : powerlib/Measurements/Three-Phase V-I Measurement  VoltageMeasurement=phase-to-ground  SetLabelV=on  LabelV=Vabc_B2300  Vpu=on  VpuLL=off  CurrentMeasurement=yes  SetLabelI=on  LabelI=Iabc_B2300  Ipu=on  Pbase=2.0e6  Vbase=2300  OutputType=Complex  PhasorSimulation=on  PSBequivalent=0
  Bus Selector : BusSelector  OutputSignals=Mechanical.Rotor speed (wm)
  Data Type Conversion : DataTypeConversion  OutDataTypeStr=double  SampleTime=0  SaturateOnIntegerOverflow=on  RndMeth=Zero
  Gain : Gain  Gain=0.9  SaturateOnIntegerOverflow=on  OutDataTypeStr=Inherit: Same as input  ParamDataTypeStr=Inherit: Same as input
  Ground : powerlib/Elements/Ground  LConnTagsString=a
  Ground1 : Ground
  Ground2 : Ground
  Logical Operator : Logic  Operator=NOT  AllPortsSameDT=off
  PF Correction Capacitor 800 kvar : powerlib/Elements/Three-Phase Series RLC Load  LConnTagsString=A|B|C  Configuration=Y (grounded)  NominalVoltage=2300  Vabc=[1e3 1e3 1e3]  Vabcp=[1e3 1e3 1e3]  NominalFrequency=60  UnbalancedPower=off  ActivePower=0  InductivePower=0  CapacitivePower=800e3  Pabc=[10e3 9e3 11e3]  QLabc=[100 90 110]  QCabc=[100 90 110]  Pabcp=[10e3 9e3 11e3]  QLabcp=[100 90 110]  QCabcp=[100 90 110]  Measurements=None  LoadType=constant Z
  Plant & Motor Protection : Subsystem  mask(Protection System){Freq=60, Max_Iinst=10, MaxI1=[ 1.1, 5 ], MaxI2I1=[ 0.4, 0.2], MinMaxV1=[ 0.9, 1.1, 0.2 ], MaxV2V1=[ 0.1, 0.1, 0.3 ], MaxVdc=[ inf, 0 ], MaxSpeed=[ 0.9, 1.1, 1 ], Delay_Protection=1}
      mask prompts: Freq "Fundamental frequency f1 (Hz):"; Max_Iinst "Instantaneous AC Overcurrent (pu):"; MaxI1 "Maximum AC Current [ I1max(pu), Delay(s) ]:"; MaxI2I1 "Maximum AC Current Unbalance [ I2/I1max(pu), Delay(s) ]"; MinMaxV1 "AC Under/Over Voltage [ V1min(pu), V1max(pu), Delay(s) ]:"; MaxV2V1 "Maximum Voltage Unbalance [ V2/V1max(pu), V0/V1max(pu), Delay(s)]:"; MaxVdc "Maximum DC Voltage  [ Vmax(V), Delay(s) ]:"; MaxSpeed "Under/Over Speed [ Speedmin (pu), Speedmax (pu), Delay(s)]:"; Delay_Protection "Start time for protection system (s):"
      mask help:
      | Protection type:
      | 1.    Instantaneous AC Overcurrent
      | 2.    AC Overcurrent (positive-sequence)
      | 3.    AC Current Unbalance
      | 4.    AC Undervoltage (positive-sequence)
      | 5.    AC Overvoltage (positive-sequence)
      | 6.    AC Voltage Unbalance (Negative-sequence)
      | 7.    AC Voltage Unbalance (Zero-sequence)
      | 8.    DC Overvoltage
      | 9.    Under Speed
      | 10.  Over Speed
      mask init:
      | a=exp(2*pi*j/3);
      | a2=a^2;
      | Max_I1=MaxI1(1);
      | Delay_I1=MaxI1(2);
      | Max_I2_I1=MaxI2I1(1);
      | Delay_I2_I1=MaxI2I1(2);
      | Min_V1=MinMaxV1(1);
      | Max_V1=MinMaxV1(2);
      | Delay_V1=MinMaxV1(3);
      | Max_V2_V1=MaxV2V1(1);
      | Max_V0_V1=MaxV2V1(2);
      | Delay_V2_V1=MaxV2V1(3);
      | Max_Vdc=MaxVdc(1);
      | Delay_Vdc=MaxVdc(2);
      | Min_Speed=MaxSpeed(1);
      | Max_Speed=MaxSpeed(2);
      | Delay_Speed=MaxSpeed(3);
  Three-Phase Breaker : powerlib/Elements/Three-Phase Breaker  InitialState=closed  SwitchA=on  SwitchB=on  SwitchC=on  SwitchTimes="[4/60  10/60]"  External=on  BreakerResistance=0.001  SnubberResistance=inf  SnubberCapacitance=inf  Measurements=None
  Trip1 : Display
  TripData : Display
  wm^2 : Fcn  Expr=u(1)^2
  A : PMIOPort  Side=Left
  B : PMIOPort  Port=2  Side=Left
  C : PMIOPort  Port=3  Side=Left
  tag scope: MotorSpeed=global
  wires:
  1.68 MW 0.93 PF 2300 V/1 -> Bus Selector/1
  Bus Selector/1 -> wm^2/1, [MotorSpeed]  "<Rotor speed (wm)>"
  wm^2/1 -> Gain/1
  [Vabc_B2300] -> Plant & Motor Protection/1(Vabc (pu))
  [Iabc_B2300] -> Plant & Motor Protection/2(Iabc (pu))
  Ground1/1 -> Plant & Motor Protection/3(Vdc (V))
  Ground2/1 -> Plant & Motor Protection/4(Reset)
  [MotorSpeed] -> Plant & Motor Protection/5(Speed (pu))
  Plant & Motor Protection/1(Trip) -> Logical Operator/1
  [Trip_Plant] -> Three-Phase Breaker/1
  Plant & Motor Protection/2(TripTime) -> Trip1/1
  Plant & Motor Protection/3(TripStatus) -> TripData/1
  Data Type Conversion/1 -> [Trip_Plant]
  Logical Operator/1 -> Data Type Conversion/1
  Gain/1 -> 1.68 MW 0.93 PF 2300 V/1
  connections:
  265 ohms/LConn1 -- 25/2.3 kV 2.5 MVA/RConn4
  Ground/LConn1 -- 265 ohms/RConn1
  A/RConn1 -- 25/2.3 kV 2.5 MVA/LConn1
  B/RConn1 -- 25/2.3 kV 2.5 MVA/LConn2
  C/RConn1 -- 25/2.3 kV 2.5 MVA/LConn3
  25/2.3 kV 2.5 MVA/RConn1 -- B2300/LConn1 -- PF Correction Capacitor 800 kvar/LConn1
  25/2.3 kV 2.5 MVA/RConn2 -- B2300/LConn2 -- PF Correction Capacitor 800 kvar/LConn2
  B2300/LConn3 -- 25/2.3 kV 2.5 MVA/RConn3 -- PF Correction Capacitor 800 kvar/LConn3
  B2300/RConn1 -- Three-Phase Breaker/LConn1
  B2300/RConn2 -- Three-Phase Breaker/LConn2
  B2300/RConn3 -- Three-Phase Breaker/LConn3
  Three-Phase Breaker/RConn1 -- 1.68 MW 0.93 PF 2300 V/LConn1 -- 200 kW/LConn1
  Three-Phase Breaker/RConn2 -- 1.68 MW 0.93 PF 2300 V/LConn2 -- 200 kW/LConn2
  Three-Phase Breaker/RConn3 -- 1.68 MW 0.93 PF 2300 V/LConn3 -- 200 kW/LConn3

== system akh_rev_project/AC System 1/Wind Turbine Protection ==
  note: Instantaneous AC Overcurrent
  note: AC Overcurrent (positive-sequence)
  note: AC Current Unbalance
  note: AC Undervoltage (positive-sequence)
  note: AC Overvoltage (positive-sequence)
  note: AC Voltage Unbalance (Negative-sequence)
  note: AC Voltage Unbalance (Zero-sequence)
  note: DC Overvoltage
  note: Under Speed
  note: Over Speed
  Ground2 : Ground
  Protection System : Subsystem  mask(Protection System){Freq=60, Max_Iinst=10, MaxI1=[ 1.1, 5 ], MaxI2I1=[ 0.4, 0.2], MinMaxV1=[ 0.75, 1.1, 0.1 ], MaxV2V1=[ 0.05, 0.05, 0.2 ], MaxVdc=[ 1900, 0.001 ], MaxSpeed=[ 0.3, 1.5, 5 ], Delay_Protection=5}
      mask prompts: Freq "Fundamental frequency f1 (Hz):"; Max_Iinst "Instantaneous AC Overcurrent (pu):"; MaxI1 "Maximum AC Current [ I1max(pu), Delay(s) ]:"; MaxI2I1 "Maximum AC Current Unbalance [ I2/I1max(pu), Delay(s) ]"; MinMaxV1 "AC Under/Over Voltage [ V1min(pu), V1max(pu), Delay(s) ]:"; MaxV2V1 "Maximum Voltage Unbalance [ V2/V1max(pu), V0/V1max(pu), Delay(s)]:"; MaxVdc "Maximum DC Voltage  [ Vmax(V), Delay(s) ]:"; MaxSpeed "Under/Over Speed [ Speedmin (pu), Speedmax (pu), Delay(s)]:"; Delay_Protection "Start time for protection system (s):"
      mask help:
      | Protection type:
      | 1.    Instantaneous AC Overcurrent
      | 2.    AC Overcurrent (positive-sequence)
      | 3.    AC Current Unbalance
      | 4.    AC Undervoltage (positive-sequence)
      | 5.    AC Overvoltage (positive-sequence)
      | 6.    AC Voltage Unbalance (Negative-sequence)
      | 7.    AC Voltage Unbalance (Zero-sequence)
      | 8.    DC Overvoltage
      | 9.    Under Speed
      | 10.  Over Speed
      mask init: same as akh_rev_project/AC System 1/Plant 2 MVA/Plant & Motor Protection
  TripData : Display
  Trip : Outport  VectorParamsAs1DForOutWhenUnconnected=off
  Trip Time : Outport  Port=2  VectorParamsAs1DForOutWhenUnconnected=off
  wires:
  Ground2/1 -> Protection System/4(Reset)
  Protection System/3(TripStatus) -> TripData/1
  [Vabc_B575] -> Protection System/1(Vabc (pu))
  [Vdc] -> Protection System/3(Vdc (V))
  [wr] -> Protection System/5(Speed (pu))
  [Iabc_B575] -> Protection System/2(Iabc (pu))
  Protection System/1(Trip) -> Trip/1
  Protection System/2(TripTime) -> Trip Time/1

== system akh_rev_project/AC System 2/Bus_1 ==
  Bus : powerlib/Measurements/Three-Phase V-I Measurement  VoltageMeasurement=phase-to-phase  SetLabelV=on  LabelV=VB_1  Vpu=off  VpuLL=off  CurrentMeasurement=yes  SetLabelI=on  LabelI=IB_1  Ipu=off  Pbase=100e6  Vbase=500e3  OutputType=Complex  PhasorSimulation=off  PSBequivalent=0
  Bus_ : powerlib/Measurements/Three-Phase V-I Measurement  VoltageMeasurement=phase-to-phase  SetLabelV=on  LabelV=V_B1  Vpu=off  VpuLL=off  CurrentMeasurement=yes  SetLabelI=on  LabelI=I_B1  Ipu=off  Pbase=100e6  Vbase=500e3  OutputType=Complex  PhasorSimulation=off  PSBequivalent=0
  Conn1 : PMIOPort  Side=Left
  Conn2 : PMIOPort  Port=2  Side=Right
  Conn3 : PMIOPort  Port=3  Side=Left
  Conn4 : PMIOPort  Port=4  Side=Right
  Conn5 : PMIOPort  Port=5  Side=Right
  Conn6 : PMIOPort  Port=6  Side=Left
  Conn7 : PMIOPort  Port=7  Side=Right
  Conn8 : PMIOPort  Port=8  Side=Right
  Conn9 : PMIOPort  Port=9  Side=Right
  connections:
  Conn6/RConn1 -- Bus_/LConn1 -- Bus/LConn3
  Bus/RConn2 -- Conn4/RConn1
  Bus_/RConn2 -- Conn8/RConn1
  Bus/LConn2 -- Bus_/LConn2 -- Conn3/RConn1
  Bus/LConn1 -- Bus_/LConn3 -- Conn1/RConn1
  Conn5/RConn1 -- Bus/RConn1
  Conn2/RConn1 -- Bus/RConn3
  Conn9/RConn1 -- Bus_/RConn1
  Conn7/RConn1 -- Bus_/RConn3

== system akh_rev_project/AC System 2/Bus_10 ==
  Bus : powerlib/Measurements/Three-Phase V-I Measurement  VoltageMeasurement=phase-to-phase  SetLabelV=on  LabelV=VB_10  Vpu=off  VpuLL=off  CurrentMeasurement=yes  SetLabelI=on  LabelI=IB_10  Ipu=off  Pbase=100e6  Vbase=500e3  OutputType=Complex  PhasorSimulation=off  PSBequivalent=0
  Bus_ : powerlib/Measurements/Three-Phase V-I Measurement  VoltageMeasurement=phase-to-phase  SetLabelV=on  LabelV=V_B10  Vpu=off  VpuLL=off  CurrentMeasurement=yes  SetLabelI=on  LabelI=I_B10  Ipu=off  Pbase=100e6  Vbase=500e3  OutputType=Complex  PhasorSimulation=off  PSBequivalent=0
  Conn1 : PMIOPort  Side=Left
  Conn2 : PMIOPort  Port=2  Side=Right
  Conn3 : PMIOPort  Port=3  Side=Left
  Conn4 : PMIOPort  Port=4  Side=Right
  Conn5 : PMIOPort  Port=5  Side=Right
  Conn6 : PMIOPort  Port=6  Side=Left
  Conn7 : PMIOPort  Port=7  Side=Right
  Conn8 : PMIOPort  Port=8  Side=Right
  Conn9 : PMIOPort  Port=9  Side=Right
  connections:
  Conn1/RConn1 -- Bus_/LConn3 -- Bus/LConn1
  Conn3/RConn1 -- Bus_/LConn2 -- Bus/LConn2
  Bus_/RConn2 -- Conn8/RConn1
  Bus/RConn2 -- Conn4/RConn1
  Bus/LConn3 -- Bus_/LConn1 -- Conn6/RConn1
  Bus_/RConn1 -- Conn7/RConn1
  Bus_/RConn3 -- Conn9/RConn1
  Bus/RConn1 -- Conn2/RConn1
  Bus/RConn3 -- Conn5/RConn1

== system akh_rev_project/AC System 2/Bus_11 ==
  Bus : powerlib/Measurements/Three-Phase V-I Measurement  VoltageMeasurement=phase-to-phase  SetLabelV=on  LabelV=VB_11  Vpu=off  VpuLL=off  CurrentMeasurement=yes  SetLabelI=on  LabelI=IB_11  Ipu=off  Pbase=100e6  Vbase=500e3  OutputType=Complex  PhasorSimulation=off  PSBequivalent=0
  Bus_ : powerlib/Measurements/Three-Phase V-I Measurement  VoltageMeasurement=phase-to-phase  SetLabelV=on  LabelV=V_B11  Vpu=off  VpuLL=off  CurrentMeasurement=yes  SetLabelI=on  LabelI=I_B11  Ipu=off  Pbase=100e6  Vbase=500e3  OutputType=Complex  PhasorSimulation=off  PSBequivalent=0
  Conn1 : PMIOPort  Side=Left
  Conn2 : PMIOPort  Port=2  Side=Right
  Conn3 : PMIOPort  Port=3  Side=Left
  Conn4 : PMIOPort  Port=4  Side=Right
  Conn5 : PMIOPort  Port=5  Side=Right
  Conn6 : PMIOPort  Port=6  Side=Left
  Conn7 : PMIOPort  Port=7  Side=Right
  Conn8 : PMIOPort  Port=8  Side=Right
  Conn9 : PMIOPort  Port=9  Side=Right
  connections:
  Bus/RConn3 -- Conn5/RConn1
  Bus/RConn1 -- Conn2/RConn1
  Bus_/RConn3 -- Conn9/RConn1
  Bus_/RConn1 -- Conn7/RConn1
  Conn6/RConn1 -- Bus_/LConn1 -- Bus/LConn3
  Bus/RConn2 -- Conn4/RConn1
  Bus_/RConn2 -- Conn8/RConn1
  Bus/LConn2 -- Bus_/LConn2 -- Conn3/RConn1
  Bus/LConn1 -- Conn1/RConn1 -- Bus_/LConn3

== system akh_rev_project/AC System 2/Bus_12 ==
  Bus : powerlib/Measurements/Three-Phase V-I Measurement  VoltageMeasurement=phase-to-phase  SetLabelV=on  LabelV=VB_12  Vpu=off  VpuLL=off  CurrentMeasurement=yes  SetLabelI=on  LabelI=IB_12  Ipu=off  Pbase=100e6  Vbase=500e3  OutputType=Complex  PhasorSimulation=off  PSBequivalent=0
  Bus_ : powerlib/Measurements/Three-Phase V-I Measurement  VoltageMeasurement=phase-to-phase  SetLabelV=on  LabelV=V_B12  Vpu=off  VpuLL=off  CurrentMeasurement=yes  SetLabelI=on  LabelI=I_B12  Ipu=off  Pbase=100e6  Vbase=500e3  OutputType=Complex  PhasorSimulation=off  PSBequivalent=0
  Conn1 : PMIOPort  Side=Left
  Conn2 : PMIOPort  Port=2  Side=Right
  Conn3 : PMIOPort  Port=3  Side=Left
  Conn4 : PMIOPort  Port=4  Side=Right
  Conn5 : PMIOPort  Port=5  Side=Right
  Conn6 : PMIOPort  Port=6  Side=Left
  Conn7 : PMIOPort  Port=7  Side=Right
  Conn8 : PMIOPort  Port=8  Side=Right
  Conn9 : PMIOPort  Port=9  Side=Right
  connections:
  Conn1/RConn1 -- Bus_/LConn3 -- Bus/LConn1
  Conn3/RConn1 -- Bus_/LConn2 -- Bus/LConn2
  Bus_/RConn2 -- Conn8/RConn1
  Bus/RConn2 -- Conn4/RConn1
  Bus/LConn3 -- Bus_/LConn1 -- Conn6/RConn1
  Bus_/RConn1 -- Conn7/RConn1
  Bus_/RConn3 -- Conn9/RConn1
  Bus/RConn1 -- Conn2/RConn1
  Bus/RConn3 -- Conn5/RConn1

== system akh_rev_project/AC System 2/Bus_13 ==
  Bus : powerlib/Measurements/Three-Phase V-I Measurement  VoltageMeasurement=phase-to-phase  SetLabelV=on  LabelV=VB_13  Vpu=off  VpuLL=off  CurrentMeasurement=yes  SetLabelI=on  LabelI=IB_13  Ipu=off  Pbase=100e6  Vbase=500e3  OutputType=Complex  PhasorSimulation=off  PSBequivalent=0
  Bus_ : powerlib/Measurements/Three-Phase V-I Measurement  VoltageMeasurement=phase-to-phase  SetLabelV=on  LabelV=V_B13_13  Vpu=off  VpuLL=off  CurrentMeasurement=yes  SetLabelI=on  LabelI=I_B13_13  Ipu=off  Pbase=100e6  Vbase=500e3  OutputType=Complex  PhasorSimulation=off  PSBequivalent=0
  Bus_1 : powerlib/Measurements/Three-Phase V-I Measurement  VoltageMeasurement=phase-to-phase  SetLabelV=on  LabelV=V_B13  Vpu=off  VpuLL=off  CurrentMeasurement=yes  SetLabelI=on  LabelI=I_B13  Ipu=off  Pbase=100e6  Vbase=500e3  OutputType=Complex  PhasorSimulation=off  PSBequivalent=0
  Conn1 : PMIOPort  Side=Left
  Conn2 : PMIOPort  Port=2  Side=Right
  Conn3 : PMIOPort  Port=3  Side=Left
  Conn4 : PMIOPort  Port=4  Side=Right
  Conn5 : PMIOPort  Port=5  Side=Right
  Conn6 : PMIOPort  Port=6  Side=Left
  Conn7 : PMIOPort  Port=7  Side=Right
  Conn8 : PMIOPort  Port=8  Side=Right
  Conn9 : PMIOPort  Port=9  Side=Right
  Conn10 : PMIOPort  Port=10  Side=Right
  Conn11 : PMIOPort  Port=11  Side=Right
  Conn12 : PMIOPort  Port=12  Side=Right
  connections:
  Bus_1/LConn1 -- Bus_/LConn3 -- Conn6/RConn1 -- Bus/LConn1
  Conn3/RConn1 -- Bus/LConn2 -- Bus_1/LConn2 -- Bus_/LConn2
  Bus_/RConn2 -- Conn8/RConn1
  Bus/RConn2 -- Conn4/RConn1
  Bus_1/LConn3 -- Bus_/LConn1 -- Conn1/RConn1 -- Bus/LConn3
  Bus_/RConn1 -- Conn7/RConn1
  Bus_/RConn3 -- Conn9/RConn1
  Conn10/RConn1 -- Bus_1/RConn1
  Conn11/RConn1 -- Bus_1/RConn2
  Conn12/RConn1 -- Bus_1/RConn3
  Conn5/RConn1 -- Bus/RConn1
  Conn2/RConn1 -- Bus/RConn3
